simulink model "Celcius_Conversion_Practice"  (R2024b)
settings: Solver=VariableStepAuto  StartTime=0.0  StopTime=10.0  RelTol=1e-3
values from neighbouring files (symbols this model uses):
  X = input(prompt)    [Temp_Conversion.m]
settings Model: Creator=Stephon Woodson  LastModifiedBy=Stephon Woodson

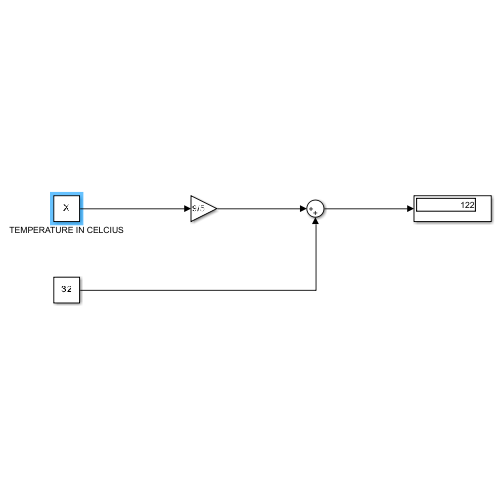
[thumbnail: Simulink's stored preview of the top-level diagram]
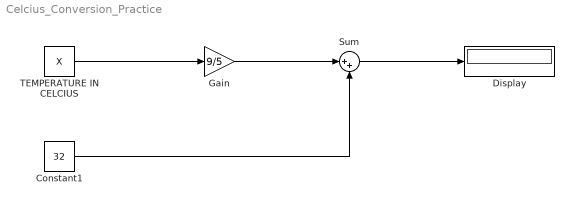
== system Celcius_Conversion_Practice ==
  Constant1 : Constant  Value=32
  Display : Display
  Gain : Gain  Gain=9/5
  Sum : Sum  Inputs=|++
  TEMPERATURE IN CELCIUS : Constant  Value=X
  wires:
  TEMPERATURE IN CELCIUS/1 -> Gain/1
  Gain/1 -> Sum/1
  Constant1/1 -> Sum/2
  Sum/1 -> Display/1
